simulink model "test"  (R2020b)
settings: Solver=VariableStepAuto  StartTime=0.0  StopTime=10.0  RelTol=1e-3
settings Model: OrderedModelArguments=off  Creator=macra  LastModifiedBy=macra

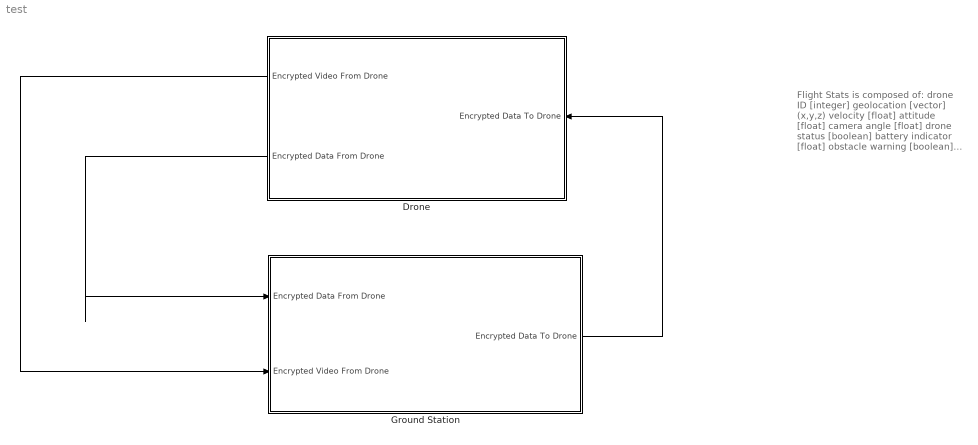
== system test ==
  note: Flight Stats is composed of:
      | drone ID			[integer]
      | geolocation         	[vector] (x,y,z)
      | velocity               	[float]
      | attitude               	[float]
      | camera angle    	[float]
      | drone status      	[boolean]
      | battery indicator 	[float]
      | obstacle warning 	[boolean]
      | ? data status        	[boolean]
  Drone : Subsystem
      settings: PortSchema="{\"entries\":[{\"content\":{\"headerSize\":26,\"margin\":15,\"minimumSpacing\":25,\"sides\":[{\"content\":{\"connectorIds\":[\"Out1\",\"Out2\"]},\"type\":\"ConnectorPlacement.EquallySpacedRectSide\",\"uuid\":\"5dbdb512-c724-4537-b423-e7f241817497\"},{\"content\":{\"connectorIds\":[\"In1\"],\"side\":\"RIGHT\"},\"type\":\"ConnectorPlacement.EquallySpacedRectSide\",\"uuid\":\"ed169a95-4211-4c22-8607-e2cdf6a6fff2\"},{\"content\":{\"connectorIds\":[],\"side\":\"TOP\"},\"type\":\"ConnectorPlacement.EquallySpacedRectSide\",\"uuid\":\"83c28233-b95d-4084-ab80-743a8fa582e0\"},{\"content\":{\"connectorIds\":[],\"side\":\"HIDDEN\"},\"type\":\"ConnectorPlacement.EquallySpacedRectSide\",\"uuid\":\"78dc0539-d843-45d4-8b50-0f9c194c2eeb\"}]},\"type\":\"ConnectorPlacement.EquallySpacedConnector\",\"uuid\":\"65b23c69-016e-4b27-94b8-7f752ac94c38\"}],\"packageUris\":[\"http://schema.mathworks.com/mf0/Connector/R2020b\"],\"version\":\"1.0\"}"
  Ground Station : Subsystem
      settings: PortSchema="{\"entries\":[{\"content\":{\"headerSize\":26,\"margin\":15,\"minimumSpacing\":25,\"sides\":[{\"content\":{\"connectorIds\":[\"In1\",\"In2\"]},\"type\":\"ConnectorPlacement.EquallySpacedRectSide\",\"uuid\":\"5dbdb512-c724-4537-b423-e7f241817497\"},{\"content\":{\"connectorIds\":[\"Out1\"],\"side\":\"RIGHT\"},\"type\":\"ConnectorPlacement.EquallySpacedRectSide\",\"uuid\":\"ed169a95-4211-4c22-8607-e2cdf6a6fff2\"},{\"content\":{\"connectorIds\":[],\"side\":\"TOP\"},\"type\":\"ConnectorPlacement.EquallySpacedRectSide\",\"uuid\":\"83c28233-b95d-4084-ab80-743a8fa582e0\"},{\"content\":{\"connectorIds\":[],\"side\":\"HIDDEN\"},\"type\":\"ConnectorPlacement.EquallySpacedRectSide\",\"uuid\":\"78dc0539-d843-45d4-8b50-0f9c194c2eeb\"}]},\"type\":\"ConnectorPlacement.EquallySpacedConnector\",\"uuid\":\"65b23c69-016e-4b27-94b8-7f752ac94c38\"}],\"packageUris\":[\"http://schema.mathworks.com/mf0/Connector/R2020b\"],\"version\":\"1.0\"}"
  wires:
  Drone/2(Encrypted Data From Drone) -> Ground Station/1(Encrypted Data From Drone)
  Drone/1(Encrypted Video From Drone) -> Ground Station/2(Encrypted Video From Drone)
  Ground Station/1(Encrypted Data To Drone) -> Drone/1(Encrypted Data To Drone)

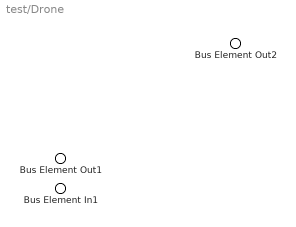
== system test/Drone ==
  Bus Element In1 : Inport  PortName=Encrypted Data To Drone
  Bus Element Out2 : Outport  PortName=Encrypted Video From Drone
  Bus Element Out1 : Outport  Port=2  PortName=Encrypted Data From Drone

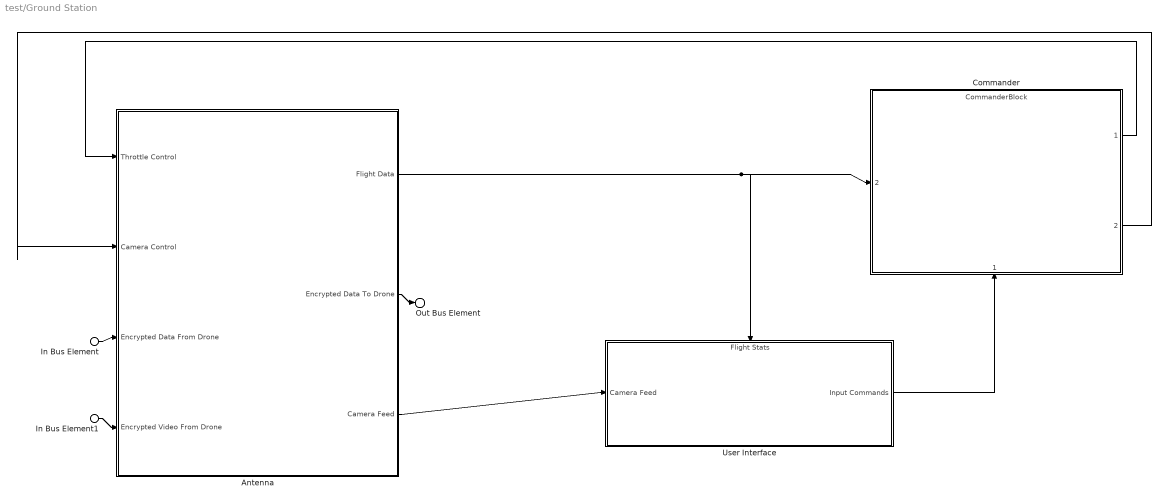
== system test/Ground Station ==
  In Bus Element : Inport  PortName=Encrypted Data From Drone
  In Bus Element1 : Inport  Port=2  PortName=Encrypted Video From Drone
  Antenna : Subsystem
      settings: PortSchema="{\"entries\":[{\"content\":{\"headerSize\":26,\"margin\":15,\"minimumSpacing\":25,\"sides\":[{\"content\":{\"connectorIds\":[\"In1\",\"In2\",\"In3\",\"In4\"]},\"type\":\"ConnectorPlacement.EquallySpacedRectSide\",\"uuid\":\"8f51257f-f627-4f58-a4af-3e0fb88ba4bc\"},{\"content\":{\"connectorIds\":[\"Out1\",\"Out3\",\"Out2\"],\"side\":\"RIGHT\"},\"type\":\"ConnectorPlacement.EquallySpacedRectSide\",\"uuid\":\"f1fa1950-8e47-40b7-8d13-b3d0804be378\"},{\"content\":{\"connectorIds\":[],\"side\":\"TOP\"},\"type\":\"ConnectorPlacement.EquallySpacedRectSide\",\"uuid\":\"7a27bdc2-dc0c-4d7e-ba2c-0c757f448581\"},{\"content\":{\"connectorIds\":[],\"side\":\"HIDDEN\"},\"type\":\"ConnectorPlacement.EquallySpacedRectSide\",\"uuid\":\"bf1e85f7-7c79-4931-85e3-188682710bd5\"}]},\"type\":\"ConnectorPlacement.EquallySpacedConnector\",\"uuid\":\"5f8c8835-300e-4f03-b548-6a322d546785\"}],\"packageUris\":[\"http://schema.mathworks.com/mf0/Connector/R2020b\"],\"version\":\"1.0\"}"
  Commander : ModelReference  ModelNameDialog=CommanderBlock  SimulationMode=Normal  ModelReferenceVersion=1.3
      settings: PortSchema="{\"entries\":[{\"content\":{\"headerSize\":38,\"margin\":15,\"minimumSpacing\":25,\"sides\":[{\"content\":{\"connectorIds\":[\"In2\"]},\"type\":\"ConnectorPlacement.EquallySpacedRectSide\",\"uuid\":\"8f51257f-f627-4f58-a4af-3e0fb88ba4bc\"},{\"content\":{\"connectorIds\":[\"Out1\",\"Out2\"],\"side\":\"RIGHT\"},\"type\":\"ConnectorPlacement.EquallySpacedRectSide\",\"uuid\":\"f1fa1950-8e47-40b7-8d13-b3d0804be378\"},{\"content\":{\"connectorIds\":[],\"side\":\"TOP\"},\"type\":\"ConnectorPlacement.EquallySpacedRectSide\",\"uuid\":\"7a27bdc2-dc0c-4d7e-ba2c-0c757f448581\"},{\"content\":{\"connectorIds\":[\"In1\"],\"side\":\"BOTTOM\"},\"type\":\"ConnectorPlacement.EquallySpacedRectSide\",\"uuid\":\"100c20a7-19a0-4abc-9a19-4a6d998db79c\"},{\"content\":{\"connectorIds\":[],\"side\":\"HIDDEN\"},\"type\":\"ConnectorPlacement.EquallySpacedRectSide\",\"uuid\":\"bf1e85f7-7c79-4931-85e3-188682710bd5\"}]},\"type\":\"ConnectorPlacement.EquallySpacedConnector\",\"uuid\":\"5f8c8835-300e-4f03-b548-6a322d546785\"}],\"packageUris\":[\"http://schema.mathworks.com/mf0/Connector/R2020b\"],\"version\":\"1.0\"}"
  User Interface : Subsystem
      settings: PortSchema="{\"entries\":[{\"content\":{\"headerSize\":26,\"margin\":15,\"minimumSpacing\":25,\"sides\":[{\"content\":{\"connectorIds\":[\"In2\"]},\"type\":\"ConnectorPlacement.EquallySpacedRectSide\",\"uuid\":\"8f51257f-f627-4f58-a4af-3e0fb88ba4bc\"},{\"content\":{\"connectorIds\":[\"Out1\"],\"side\":\"RIGHT\"},\"type\":\"ConnectorPlacement.EquallySpacedRectSide\",\"uuid\":\"f1fa1950-8e47-40b7-8d13-b3d0804be378\"},{\"content\":{\"connectorIds\":[\"In1\"],\"side\":\"TOP\"},\"type\":\"ConnectorPlacement.EquallySpacedRectSide\",\"uuid\":\"7a27bdc2-dc0c-4d7e-ba2c-0c757f448581\"},{\"content\":{\"connectorIds\":[],\"side\":\"HIDDEN\"},\"type\":\"ConnectorPlacement.EquallySpacedRectSide\",\"uuid\":\"bf1e85f7-7c79-4931-85e3-188682710bd5\"}]},\"type\":\"ConnectorPlacement.EquallySpacedConnector\",\"uuid\":\"5f8c8835-300e-4f03-b548-6a322d546785\"}],\"packageUris\":[\"http://schema.mathworks.com/mf0/Connector/R2020b\"],\"version\":\"1.0\"}"
  Out Bus Element : Outport  PortName=Encrypted Data To Drone
  wires:
  Antenna/2(Camera Feed) -> User Interface/2(Camera Feed)
  In Bus Element/1 -> Antenna/3(Encrypted Data From Drone)
  Antenna/3(Encrypted Data To Drone) -> Out Bus Element/1
  In Bus Element1/1 -> Antenna/4(Encrypted Video From Drone)
  Antenna/1(Flight Data) -> User Interface/1(Flight Stats), Commander/2
  User Interface/1(Input Commands) -> Commander/1
  Commander/1 -> Antenna/1(Throttle Control)
  Commander/2 -> Antenna/2(Camera Control)

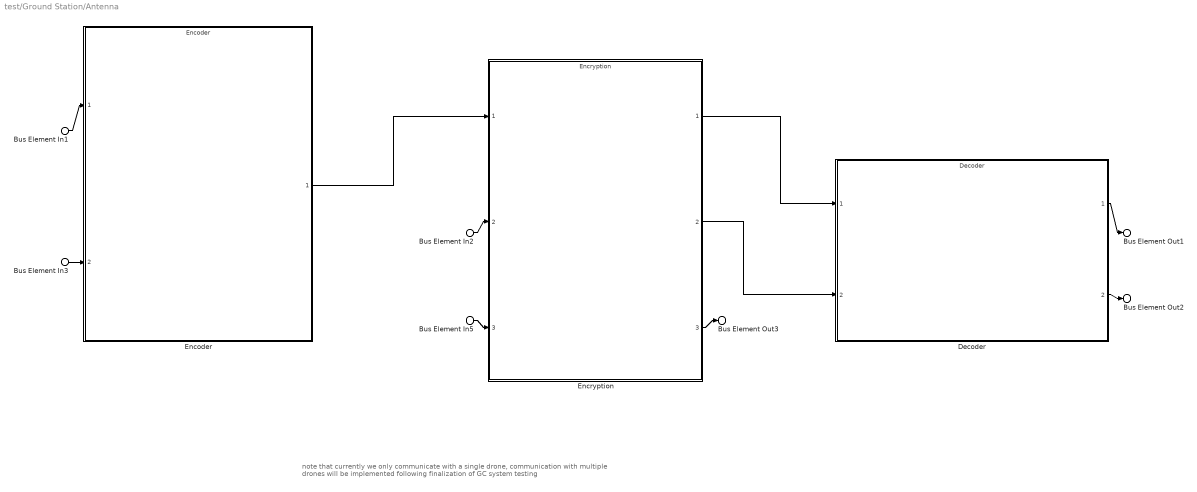
== system test/Ground Station/Antenna ==
  note: note that currently we only communicate with a single drone, communication with multiple drones will be implemented following finalization of GC system testing
  Bus Element In1 : Inport  PortName=Throttle Control
  Bus Element In3 : Inport  Port=2  PortName=Camera Control
  Bus Element In2 : Inport  Port=3  PortName=Encrypted Data From Drone
  Bus Element In5 : Inport  Port=4  PortName=Encrypted Video From Drone
  Decoder : ModelReference  ModelNameDialog=Decoder  SimulationMode=Normal  ModelReferenceVersion=1.10
      settings: PortSchema="{\"entries\":[{\"content\":{\"headerSize\":38,\"margin\":15,\"minimumSpacing\":25,\"sides\":[{\"content\":{\"connectorIds\":[\"In1\",\"In2\"]},\"type\":\"ConnectorPlacement.EquallySpacedRectSide\",\"uuid\":\"8f51257f-f627-4f58-a4af-3e0fb88ba4bc\"},{\"content\":{\"connectorIds\":[\"Out1\",\"Out2\"],\"side\":\"RIGHT\"},\"type\":\"ConnectorPlacement.EquallySpacedRectSide\",\"uuid\":\"f1fa1950-8e47-40b7-8d13-b3d0804be378\"},{\"content\":{\"connectorIds\":[],\"side\":\"TOP\"},\"type\":\"ConnectorPlacement.EquallySpacedRectSide\",\"uuid\":\"7a27bdc2-dc0c-4d7e-ba2c-0c757f448581\"},{\"content\":{\"connectorIds\":[],\"side\":\"HIDDEN\"},\"type\":\"ConnectorPlacement.EquallySpacedRectSide\",\"uuid\":\"bf1e85f7-7c79-4931-85e3-188682710bd5\"}]},\"type\":\"ConnectorPlacement.EquallySpacedConnector\",\"uuid\":\"5f8c8835-300e-4f03-b548-6a322d546785\"}],\"packageUris\":[\"http://schema.mathworks.com/mf0/Connector/R2020b\"],\"version\":\"1.0\"}"
  Encoder : ModelReference  ModelNameDialog=Encoder.slx  SimulationMode=Normal  ModelReferenceVersion=1.7
      settings: PortSchema="{\"entries\":[{\"content\":{\"headerSize\":38,\"margin\":15,\"minimumSpacing\":25,\"sides\":[{\"content\":{\"connectorIds\":[\"In1\",\"In2\"]},\"type\":\"ConnectorPlacement.EquallySpacedRectSide\",\"uuid\":\"8f51257f-f627-4f58-a4af-3e0fb88ba4bc\"},{\"content\":{\"connectorIds\":[\"Out1\"],\"side\":\"RIGHT\"},\"type\":\"ConnectorPlacement.EquallySpacedRectSide\",\"uuid\":\"f1fa1950-8e47-40b7-8d13-b3d0804be378\"},{\"content\":{\"connectorIds\":[],\"side\":\"TOP\"},\"type\":\"ConnectorPlacement.EquallySpacedRectSide\",\"uuid\":\"7a27bdc2-dc0c-4d7e-ba2c-0c757f448581\"},{\"content\":{\"connectorIds\":[],\"side\":\"HIDDEN\"},\"type\":\"ConnectorPlacement.EquallySpacedRectSide\",\"uuid\":\"bf1e85f7-7c79-4931-85e3-188682710bd5\"}]},\"type\":\"ConnectorPlacement.EquallySpacedConnector\",\"uuid\":\"5f8c8835-300e-4f03-b548-6a322d546785\"}],\"packageUris\":[\"http://schema.mathworks.com/mf0/Connector/R2020b\"],\"version\":\"1.0\"}"
  Encryption : ModelReference  ModelNameDialog=Encryption  SimulationMode=Normal  ModelReferenceVersion=1.3
      settings: PortSchema="{\"entries\":[{\"content\":{\"headerSize\":38,\"margin\":15,\"minimumSpacing\":25,\"sides\":[{\"content\":{\"connectorIds\":[\"In1\",\"In2\",\"In3\"]},\"type\":\"ConnectorPlacement.EquallySpacedRectSide\",\"uuid\":\"8f51257f-f627-4f58-a4af-3e0fb88ba4bc\"},{\"content\":{\"connectorIds\":[\"Out1\",\"Out2\",\"Out3\"],\"side\":\"RIGHT\"},\"type\":\"ConnectorPlacement.EquallySpacedRectSide\",\"uuid\":\"f1fa1950-8e47-40b7-8d13-b3d0804be378\"},{\"content\":{\"connectorIds\":[],\"side\":\"TOP\"},\"type\":\"ConnectorPlacement.EquallySpacedRectSide\",\"uuid\":\"7a27bdc2-dc0c-4d7e-ba2c-0c757f448581\"},{\"content\":{\"connectorIds\":[],\"side\":\"HIDDEN\"},\"type\":\"ConnectorPlacement.EquallySpacedRectSide\",\"uuid\":\"bf1e85f7-7c79-4931-85e3-188682710bd5\"}]},\"type\":\"ConnectorPlacement.EquallySpacedConnector\",\"uuid\":\"5f8c8835-300e-4f03-b548-6a322d546785\"}],\"packageUris\":[\"http://schema.mathworks.com/mf0/Connector/R2020b\"],\"version\":\"1.0\"}"
  Bus Element Out1 : Outport  PortName=Flight Data
  Bus Element Out2 : Outport  Port=2  PortName=Camera Feed
  Bus Element Out3 : Outport  Port=3  PortName=Encrypted Data To Drone
  wires:
  Bus Element In2/1 -> Encryption/2
  Bus Element In5/1 -> Encryption/3
  Encryption/3 -> Bus Element Out3/1
  Encryption/1 -> Decoder/1
  Encryption/2 -> Decoder/2
  Decoder/2 -> Bus Element Out2/1
  Decoder/1 -> Bus Element Out1/1
  Encoder/1 -> Encryption/1
  Bus Element In1/1 -> Encoder/1
  Bus Element In3/1 -> Encoder/2

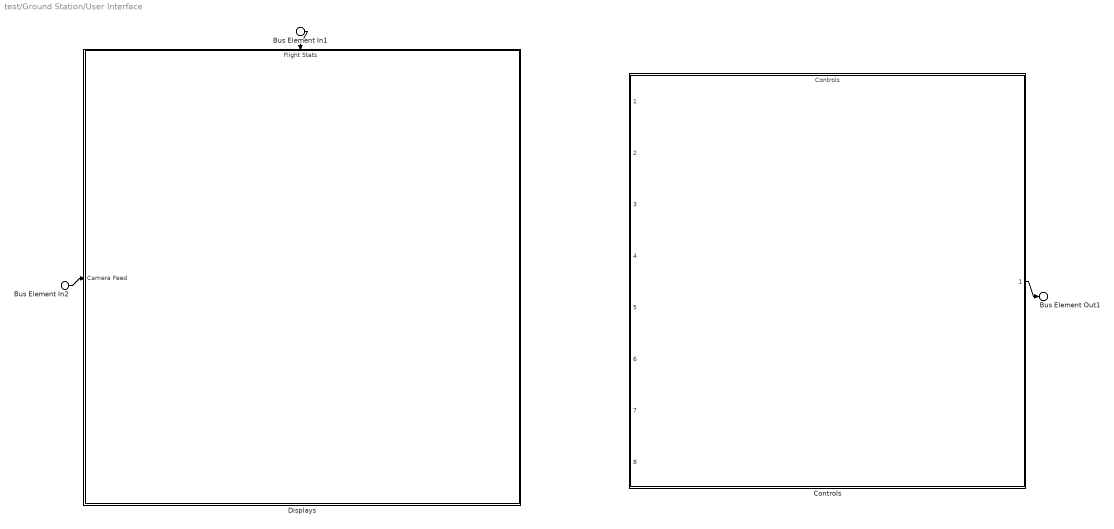
== system test/Ground Station/User Interface ==
  Bus Element In1 : Inport  PortName=Flight Stats
  Bus Element In2 : Inport  Port=2  PortName=Camera Feed
  Controls : ModelReference  ModelNameDialog=Controls  SimulationMode=Normal  ModelReferenceVersion=1.5
      settings: PortSchema="{\"entries\":[{\"content\":{\"headerSize\":38,\"margin\":15,\"minimumSpacing\":25,\"sides\":[{\"content\":{\"connectorIds\":[\"In1\",\"In2\",\"In3\",\"In4\",\"In5\",\"In6\",\"In7\",\"In8\"]},\"type\":\"ConnectorPlacement.EquallySpacedRectSide\",\"uuid\":\"8f51257f-f627-4f58-a4af-3e0fb88ba4bc\"},{\"content\":{\"connectorIds\":[\"Out1\"],\"side\":\"RIGHT\"},\"type\":\"ConnectorPlacement.EquallySpacedRectSide\",\"uuid\":\"f1fa1950-8e47-40b7-8d13-b3d0804be378\"},{\"content\":{\"connectorIds\":[],\"side\":\"TOP\"},\"type\":\"ConnectorPlacement.EquallySpacedRectSide\",\"uuid\":\"7a27bdc2-dc0c-4d7e-ba2c-0c757f448581\"},{\"content\":{\"connectorIds\":[],\"side\":\"HIDDEN\"},\"type\":\"ConnectorPlacement.EquallySpacedRectSide\",\"uuid\":\"bf1e85f7-7c79-4931-85e3-188682710bd5\"}]},\"type\":\"ConnectorPlacement.EquallySpacedConnector\",\"uuid\":\"5f8c8835-300e-4f03-b548-6a322d546785\"}],\"packageUris\":[\"http://schema.mathworks.com/mf0/Connector/R2020b\"],\"version\":\"1.0\"}"
  Displays : Subsystem
      settings: PortSchema="{\"entries\":[{\"content\":{\"headerSize\":26,\"margin\":15,\"minimumSpacing\":25,\"sides\":[{\"content\":{\"connectorIds\":[\"In1\"]},\"type\":\"ConnectorPlacement.EquallySpacedRectSide\",\"uuid\":\"8f51257f-f627-4f58-a4af-3e0fb88ba4bc\"},{\"content\":{\"connectorIds\":[],\"side\":\"RIGHT\"},\"type\":\"ConnectorPlacement.EquallySpacedRectSide\",\"uuid\":\"f1fa1950-8e47-40b7-8d13-b3d0804be378\"},{\"content\":{\"connectorIds\":[\"In2\"],\"side\":\"TOP\"},\"type\":\"ConnectorPlacement.EquallySpacedRectSide\",\"uuid\":\"7a27bdc2-dc0c-4d7e-ba2c-0c757f448581\"},{\"content\":{\"connectorIds\":[],\"side\":\"HIDDEN\"},\"type\":\"ConnectorPlacement.EquallySpacedRectSide\",\"uuid\":\"bf1e85f7-7c79-4931-85e3-188682710bd5\"}]},\"type\":\"ConnectorPlacement.EquallySpacedConnector\",\"uuid\":\"5f8c8835-300e-4f03-b548-6a322d546785\"}],\"packageUris\":[\"http://schema.mathworks.com/mf0/Connector/R2020b\"],\"version\":\"1.0\"}"
  Bus Element Out1 : Outport  PortName=Input Commands
  wires:
  Bus Element In1/1 -> Displays/2(Flight Stats)
  Bus Element In2/1 -> Displays/1(Camera Feed)
  Controls/1 -> Bus Element Out1/1

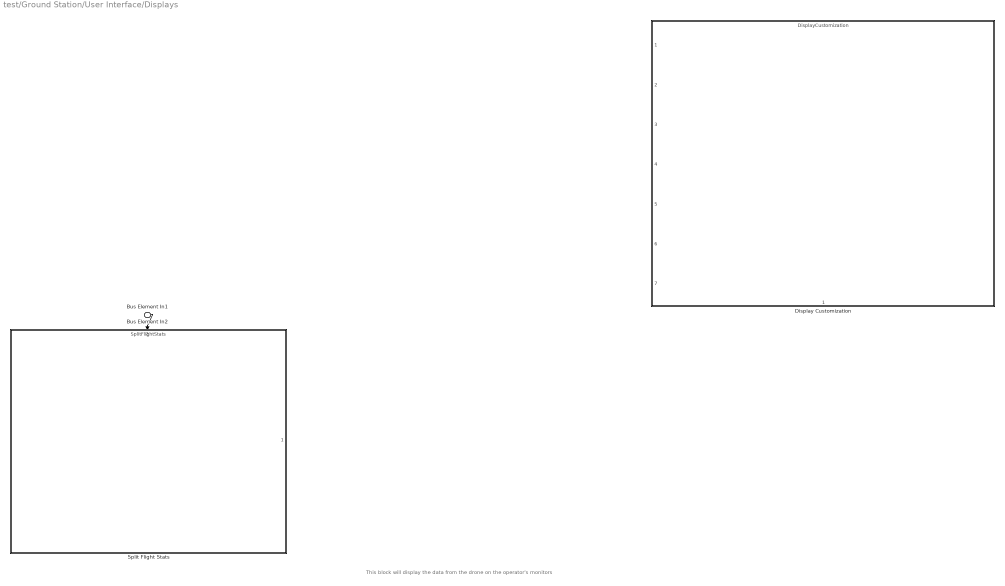
== system test/Ground Station/User Interface/Displays ==
  note: This block will display the data from the drone on the operator's monitors
  Bus Element In2 : Inport  PortName=Camera Feed
  Bus Element In1 : Inport  Port=2  PortName=Flight Stats
  Display Customization : ModelReference  ModelNameDialog=DisplayCustomization  SimulationMode=Normal  ModelReferenceVersion=1.9
      settings: PortSchema="{\"entries\":[{\"content\":{\"headerSize\":38,\"margin\":15,\"minimumSpacing\":25,\"sides\":[{\"content\":{\"connectorIds\":[\"In1\",\"In2\",\"In3\",\"In4\",\"In5\",\"In6\",\"In7\"]},\"type\":\"ConnectorPlacement.EquallySpacedRectSide\",\"uuid\":\"8f51257f-f627-4f58-a4af-3e0fb88ba4bc\"},{\"content\":{\"connectorIds\":[],\"side\":\"RIGHT\"},\"type\":\"ConnectorPlacement.EquallySpacedRectSide\",\"uuid\":\"f1fa1950-8e47-40b7-8d13-b3d0804be378\"},{\"content\":{\"connectorIds\":[],\"side\":\"TOP\"},\"type\":\"ConnectorPlacement.EquallySpacedRectSide\",\"uuid\":\"7a27bdc2-dc0c-4d7e-ba2c-0c757f448581\"},{\"content\":{\"connectorIds\":[\"Out1\"],\"side\":\"BOTTOM\"},\"type\":\"ConnectorPlacement.EquallySpacedRectSide\",\"uuid\":\"32250273-8758-4d14-a54c-b4912de856f8\"},{\"content\":{\"connectorIds\":[],\"side\":\"HIDDEN\"},\"type\":\"ConnectorPlacement.EquallySpacedRectSide\",\"uuid\":\"bf1e85f7-7c79-4931-85e3-188682710bd5\"}]},\"type\":\"ConnectorPlacement.EquallySpacedConnector\",\"uuid\":\"5f8c8835-300e-4f03-b548-6a322d546785\"}],\"packageUris\":[\"http://schema.mathworks.com/mf0/Connector/R2020b\"],\"version\":\"1.0\"}"
  Split Flight Stats : ModelReference  ModelNameDialog=SplitFlightStats  SimulationMode=Normal  ModelReferenceVersion=1.12
      settings: PortSchema="{\"entries\":[{\"content\":{\"headerSize\":38,\"margin\":15,\"minimumSpacing\":25,\"sides\":[{\"content\":{\"connectorIds\":[]},\"type\":\"ConnectorPlacement.EquallySpacedRectSide\",\"uuid\":\"f1942fcd-7656-491b-a1c1-0009704286d0\"},{\"content\":{\"connectorIds\":[\"In1\"],\"side\":\"RIGHT\"},\"type\":\"ConnectorPlacement.EquallySpacedRectSide\",\"uuid\":\"8c462db5-e755-4394-aa25-af0391ddb18d\"},{\"content\":{\"connectorIds\":[\"In2\"],\"side\":\"TOP\"},\"type\":\"ConnectorPlacement.EquallySpacedRectSide\",\"uuid\":\"153622cc-35b1-41b1-bad2-e93a3c840798\"},{\"content\":{\"connectorIds\":[],\"side\":\"HIDDEN\"},\"type\":\"ConnectorPlacement.EquallySpacedRectSide\",\"uuid\":\"1ba78c84-130a-4200-a78a-ba538d9bc02e\"}]},\"type\":\"ConnectorPlacement.EquallySpacedConnector\",\"uuid\":\"db09f390-11f3-4188-aba1-207abe1801fd\"}],\"packageUris\":[\"http://schema.mathworks.com/mf0/Connector/R2020b\"],\"version\":\"1.0\"}"
  wires:
  Bus Element In1/1 -> Split Flight Stats/2
